simulink model "belt_driven_ergometer"  (R2019b)
settings: Solver=VariableStepAuto  StartTime=0.0  StopTime=10.0  RelTol=1e-3
InitFcn:
  | Kt=0.21
  | rm=0.0135
  | rf=0.15
  | Jm=5.3e-5
  | Jf=2.57e-2
  | Jeq=2.62e-4
  | Jp=5.2e-3
  | Kbelt=8312.1
  | Bbelt=5.96
  | K1=15791
  | K2=251.33
  | N=11.11
  | Ka=2.52e-2
  | Kp=1.664
  | Ki=26.1382
undefined symbols (not defined in the file or in its folder): f, Jeqe, Kte
libraries: powerlib x19, powerlib_extras x3, powerlib_meascontrol x2, simulink x2
settings Model: Creator=李瑾年  LastModifiedBy=李瑾年

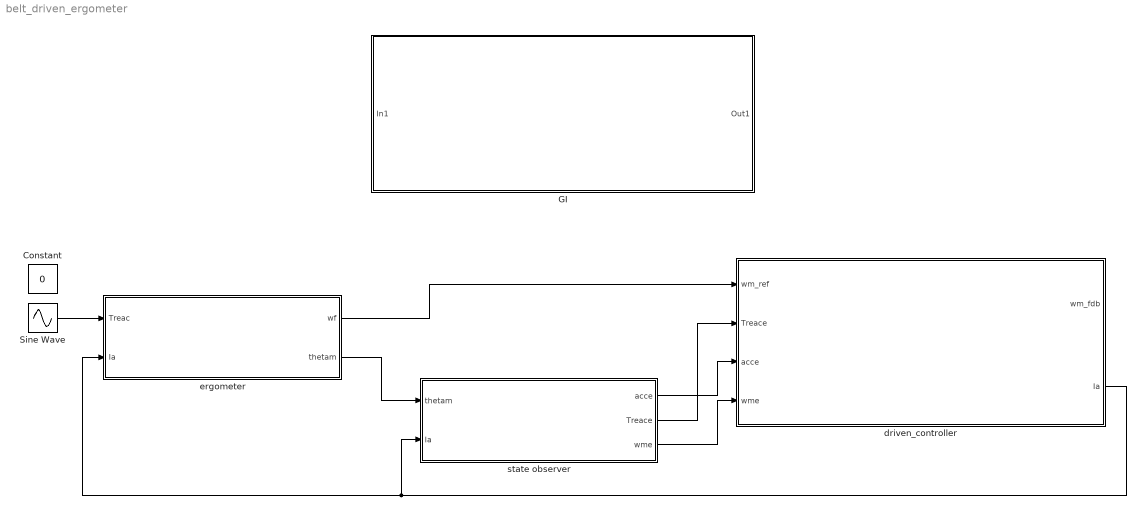
== system belt_driven_ergometer ==
  Constant : Constant  Value=0
  GI : Subsystem
  Sine Wave : Sin  Amplitude=0.5  Bias=-0.5  Frequency=2*pi*f  SampleTime=0
  driven_controller : Subsystem
  ergometer : Subsystem
  state observer : Subsystem
  wires:
  ergometer/1(wf) -> driven_controller/1(wm_ref)
  ergometer/2("thetam  ") -> state observer/1(thetam)
  state observer/2(" Treace ") -> driven_controller/2(Treace)
  state observer/1(" acce") -> driven_controller/3(acce)
  state observer/3(" wme") -> driven_controller/4(wme)
  driven_controller/2(Ia) -> ergometer/2(Ia), state observer/2(Ia)
  Sine Wave/1 -> ergometer/1(Treac)

== system belt_driven_ergometer/GI ==
  In1 : Inport
  Gain3 : Gain  Gain=N*Kt
  Qi Fcn : TransferFcn  Numerator=[15791]  Denominator=[251.33 15791]
  Qo Fcn1 : TransferFcn  Denominator=[0.05 1]
  Sum2 : Sum  Inputs=|+-
  Transfer Fcn : TransferFcn  Numerator=[K1]  Denominator=[1 K2 K1]
  Transfer Fcn1 : TransferFcn  Numerator=[K2 K1]  Denominator=[1 K2 K1]
  phai_I : TransferFcn  Numerator=[Jf rf^2*Bbelt rf^2*Kbelt]  Denominator=[Jp rf^2*Bbelt rf^2*Kbelt]
  Out1 : Outport
  wires:
  Transfer Fcn/1 -> phai_I/1
  Gain3/1 -> Qo Fcn1/1
  Sum2/1 -> Gain3/1  "a"
  Qi Fcn/1 -> Sum2/2
  phai_I/1 -> Sum2/1
  Qo Fcn1/1 -> Out1/1
  In1/1 -> Transfer Fcn1/1, Transfer Fcn/1

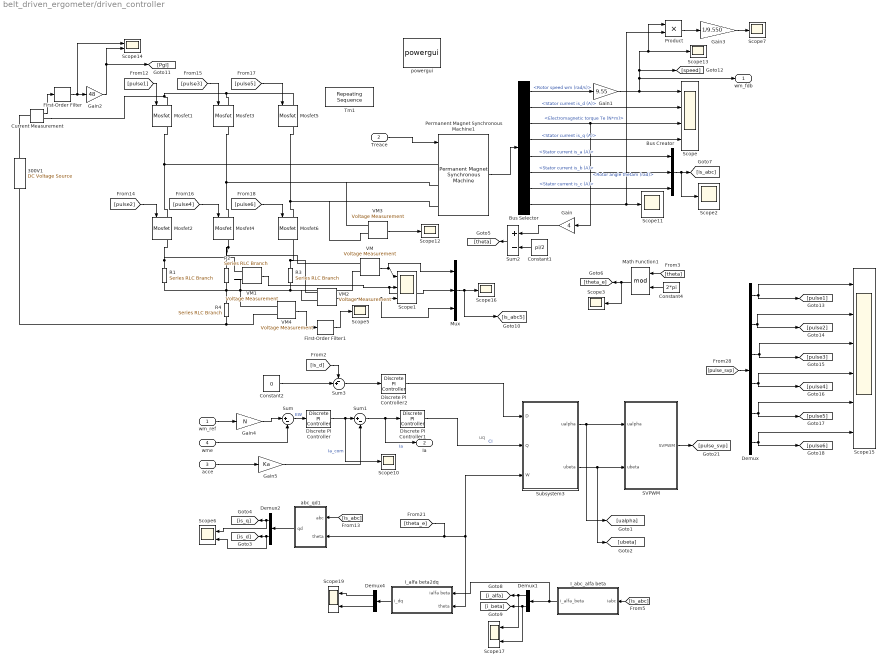
== system belt_driven_ergometer/driven_controller ==
  note: uq
  wm_ref : Inport
  Treace : Inport  Port=2
  acce : Inport  Port=3
  wme : Inport  Port=4
  300V1 : powerlib/Electrical Sources/DC Voltage Source  Amplitude=300  Measurements=Voltage
  Bus Creator : BusCreator  Inputs=3
  Bus Selector : BusSelector  OutputSignals=Rotor speed wm (rad/s),Stator current is_d (A),Rotor angle thetam (rad),Stator current is_q (A),Stator current is_a (A),Stator current is_b (A),Stator current is_c (A),Electromagnetic torque Te (N*m)
  Constant1 : Constant  Value=pi/2
  Constant2 : Constant  Value=0
  Constant4 : Constant  Value=2*pi
  Current Measurement : powerlib/Measurements/Current Measurement  PhasorSimulation=off  OutputType=Complex  PSBequivalent=0
  Demux : Demux  Outputs=6
  Demux1 : Demux  Outputs=2
  Demux2 : Demux  Outputs=2
  Demux4 : Demux  Outputs=2
  Discrete PI Controller : powerlib_extras/Discrete  Control Blocks/Discrete PI Controller  Kp=Kp  Ki=Ki  Par_Limits=[500 -500]  Init=0  Ts=50e-6
      settings: SourceProductName=Simscape Electrical
  Discrete PI Controller1 : powerlib_extras/Discrete  Control Blocks/Discrete PI Controller  Kp=50  Ki=1000  Par_Limits=[1000 -1000]  Init=0  Ts=50e-6
      settings: SourceProductName=Simscape Electrical
  Discrete PI Controller2 : powerlib_extras/Discrete  Control Blocks/Discrete PI Controller  Kp=50  Ki=1000  Par_Limits=[1000 -1000]  Init=0  Ts=50e-6
      settings: SourceProductName=Simscape Electrical
  First-Order Filter : powerlib_meascontrol/Filters/First-Order Filter  FilterType=Lowpass  Tc=0.005  Ts=5e-6  Initialize=off  Vac_Init=[0, 0, 60]  Vdc_Init=0  PlotResponse=off  FreqRange="[0,  200,  1]"
      settings: SourceProductName=Simscape Power Systems
  First-Order Filter1 : powerlib_meascontrol/Filters/First-Order Filter  FilterType=Lowpass  Tc=0.005  Ts=5e-6  Initialize=off  Vac_Init=[0, 0, 60]  Vdc_Init=0  PlotResponse=off  FreqRange="[0,  200,  1]"
      settings: SourceProductName=Simscape Power Systems
  Gain : Gain  Gain=4
  Gain1 : Gain  Gain=9.55
  Gain2 : Gain  Gain=48
  Gain3 : Gain  Gain=1/9.550
  Gain4 : Gain  Gain=N
  Gain5 : Gain  Gain=Ka
  I_abc_alfa beta : Subsystem
  I_alfa beta2dq : Subsystem
  Math Function1 : Math  Operator=mod  SaturateOnIntegerOverflow=on
  Mosfet{1..6} (6 alike) : powerlib/Power Electronics/Mosfet  Ron=0.1  Lon=0  Rd=0.01  Vfd=0  IC=0  Rs=1e5  Cs=inf  Measurements=on
  Mux : Mux  Inputs=3
  Permanent Magnet Synchronous Machine1 : powerlib/Machines/Permanent Magnet Synchronous Machine  NbPhases=3  FluxDistribution=Sinusoidal  RotorType=Round  MechanicalLoad=Torque Tm  PresetModel=No  ShowDetailedParameters=on  MeasurementBus=off  Resistance=0.033  Inductance=8.5e-3  dqInductances=[0.02682 0.02682]  La=0.000805  MachineConstant=Torque Constant (N.m / A_peak)  Flux=0.13847  VoltageCst=100.4591  TorqueCst=0.83079  Flat=120  Mechanical=[0.0001 0.0008 4]  PolePairs=4  InitialConditions=[0,0, 0,0]  InitialConditions5ph=[0 0 0 0 0 0]  RefAngle=90 degrees behind phase A axis (modified Park)  IterativeDiscreteModel=Trapezoidal non iterative  TsBlock=-1  TsPowergui=0
      settings: SourceProductName=Simscape Power Systems
  Product : Product
  R1 : powerlib/Elements/Series RLC Branch  LConnTagsString=__new0  RConnTagsString=__new0  BranchType=R  Resistance=0.003  Inductance=1e-3  SetiL0=off  InitialCurrent=0  Capacitance=1e-6  Setx0=off  InitialVoltage=0  Measurements=None
  R2 : powerlib/Elements/Series RLC Branch  LConnTagsString=__new0  RConnTagsString=__new0  BranchType=R  Resistance=0.003  Inductance=1e-3  SetiL0=off  InitialCurrent=0  Capacitance=1e-6  Setx0=off  InitialVoltage=0  Measurements=None
  R3 : powerlib/Elements/Series RLC Branch  LConnTagsString=__new0  RConnTagsString=__new0  BranchType=R  Resistance=0.003  Inductance=1e-3  SetiL0=off  InitialCurrent=0  Capacitance=1e-6  Setx0=off  InitialVoltage=0  Measurements=None
  R4 : powerlib/Elements/Series RLC Branch  LConnTagsString=__new0  RConnTagsString=__new0  BranchType=R  Resistance=0.002  Inductance=1e-3  SetiL0=off  InitialCurrent=0  Capacitance=1e-6  Setx0=off  InitialVoltage=0  Measurements=None
  SVPWM : Subsystem
  Scope : Scope  NumInputPorts=4
  Scope1 : Scope  NumInputPorts=3
  Scope{2..3,5,7,10..13,16} (9 alike) : Scope
  Scope{6,14,17,19} (4 alike) : Scope  NumInputPorts=2
  Scope15 : Scope  NumInputPorts=6
  Subsystem3 : Subsystem
  Sum : Sum  Inputs=|+-
  Sum1 : Sum  Inputs=|+-
  Sum2 : Sum  Inputs=+-  SaturateOnIntegerOverflow=on  InputSameDT=on  OutDataTypeStr=Inherit: Same as first input
  Sum3 : Sum  Inputs=-+|
  Tm1 : simulink/Sources/Repeating Sequence  rep_seq_t="[0  0.3    ]"  rep_seq_y="[ 40  70 ]"
  VM{,1..4} (5 alike) : powerlib/Measurements/Voltage Measurement  PhasorSimulation=off  OutputType=Complex  PSBequivalent=0
  abc_qd1 : Subsystem
  powergui : powerlib/powergui  SimulationMode=Discrete  SampleTime=5e-6  frequency=60  Iterations=50  frequencyindice=0  Pbase=100e6  ErrMax=1e-4  UnitsV=kV  UnitsW=MW  buscounter=0  FunctionMessages=off  echomessages=off  EnableUseOfTLC=off  CurrentSourceSwitches=off  DisableSnubberDevices=off  DisableRonSwitches=off  DisableVfSwitches=off  DisplayEquations=off  AutomaticDiscreteSolvers=off  SolverType=Tustin  Interpol=off  ExternalGateDelay=off  methode=off  Ts=0  x0status=blocks  SPID=off  SwTol=0  HookPort=off  NonlinearTolerance=1e-4  nMaxIteration=100  ContinueOnMaxIteration=off  RestoreLinks=warning  ResistiveCurrentMeasurement=off  Frange=[0:2:500]  Ylog=off  Xlog=on  ShowGrid=off  save=off  variable=ZData  structure=0  ZoomFFT=on  StartTime=0.0  cycles=1  DisplayStyle=1  fundamental=60  FreqAxis=off  MaxFrequency=1000  frequencyindicesteady=1  RmsSteady=1  display=off
  wm_fdb : Outport
  Ia : Outport  Port=2
  wires:
  I_alfa beta2dq/1(i_dq) -> Demux4/1
  abc_qd1/1(qd) -> Demux2/1
  Product/1 -> Gain3/1
  [pulse4] -> Mosfet4/1
  [pulse5] -> Mosfet5/1
  VM2/1 -> Mux/3, Scope1/3
  [pulse2] -> Mosfet2/1
  [pulse3] -> Mosfet3/1
  Permanent Magnet Synchronous Machine1/1 -> Bus Selector/1
  Demux1/2 -> [i_beta], Scope17/2
  Demux/3 -> [pulse3], Scope15/3
  Demux4/2 -> Scope19/2
  [pulse1] -> Mosfet1/1
  VM1/1 -> Mux/2, Scope1/2
  First-Order Filter1/1 -> Scope5/1
  Bus Selector/8 -> Product/2, Scope11/1  "<Electromagnetic torque Te (N*m)>"
  VM3/1 -> Scope12/1
  Discrete PI Controller1/1 -> Subsystem3/2(Q)  "CI"
  Demux/2 -> [pulse2], Scope15/2
  Subsystem3/2(ubeta) -> [ubeta], SVPWM/2(ubeta)
  [theta_e] -> I_alfa beta2dq/2(theta), Subsystem3/3(W), abc_qd1/2(theta)
  Subsystem3/1(ualpha) -> [ualpha], SVPWM/1(ualpha)
  [pulse6] -> Mosfet6/1
  Demux/4 -> [pulse4], Scope15/4
  Bus Creator/1 -> Scope2/1, [is_abc]
  Mux/1 -> [is_abcS], Scope16/1
  Bus Selector/4 -> Scope/4  "<Stator current is_q (A)>"
  wme/1 -> Sum/2
  Demux1/1 -> [i_alfa], Scope17/1
  [is_d] -> Sum3/1
  [is_abc] -> I_abc_alfa beta/1(iabc)
  VM/1 -> Mux/1, Scope1/1
  I_abc_alfa beta/1(i_alfa_beta) -> I_alfa beta2dq/1(ialfa beta), Demux1/1
  Demux/1 -> [pulse1], Scope15/1
  Gain2/1 -> [Pgl], Scope14/2
  Current Measurement/1 -> First-Order Filter/1
  Demux4/1 -> Scope19/1
  SVPWM/1(SVPWM) -> [pulse_svp]
  VM4/1 -> First-Order Filter1/1
  Gain3/1 -> Scope7/1
  First-Order Filter/1 -> Scope14/1, Gain2/1
  Math Function1/1 -> Scope3/1, [theta_e]
  Bus Selector/6 -> Bus Creator/2  "<Stator current is_b (A)>"
  Demux/6 -> [pulse6], Scope15/6
  Constant4/1 -> Math Function1/2
  Sum2/1 -> [theta]
  Demux2/2 -> Scope6/2, [is_d]
  Sum3/1 -> Discrete PI Controller2/1
  Bus Selector/2 -> Scope/2  "<Stator current is_d (A)>"
  Gain1/1 -> Scope/1, Product/1, Scope13/1, [speed], wm_fdb/1
  [theta] -> Math Function1/1
  Demux2/1 -> Scope6/1, [is_q]
  [is_abc] -> abc_qd1/1(abc)
  Sum1/1 -> Ia/1, Discrete PI Controller1/1  "Ia"
  Constant2/1 -> Sum3/2
  Bus Selector/5 -> Bus Creator/1  "<Stator current is_a (A)>"
  [pulse_svp] -> Demux/1
  Bus Selector/3 -> Gain/1, Scope/3  "<Rotor angle thetam (rad)>"
  Gain5/1 -> Sum1/2
  Discrete PI Controller/1 -> Scope10/1, Sum1/1  "Ia_com"
  Constant1/1 -> Sum2/2
  Bus Selector/1 -> Gain1/1  "<Rotor speed wm (rad/s)>"
  Bus Selector/7 -> Bus Creator/3  "<Stator current is_c (A)>"
  Discrete PI Controller2/1 -> Subsystem3/1(D)
  Gain/1 -> Sum2/1
  Sum/1 -> Discrete PI Controller/1  "EW"
  Demux/5 -> [pulse5], Scope15/5
  Treace/1 -> Permanent Magnet Synchronous Machine1/1
  wm_ref/1 -> Gain4/1
  Gain4/1 -> Sum/1
  acce/1 -> Gain5/1
  connections:
  VM4/LConn2 -- R4/RConn1 -- 300V1/LConn1
  Mosfet4/RConn1 -- VM/LConn1 -- R2/LConn1
  R3/RConn1 -- R1/RConn1 -- R4/LConn1 -- R2/RConn1 -- VM4/LConn1 -- VM1/LConn2 -- VM2/LConn2 -- VM/LConn2
  Mosfet6/LConn1 -- Mosfet5/RConn1 -- Permanent Magnet Synchronous Machine1/LConn3 -- VM3/LConn2
  Current Measurement/RConn1 -- Mosfet1/LConn1 -- Mosfet5/LConn1 -- Mosfet3/LConn1
  R1/LConn1 -- Mosfet2/RConn1 -- VM1/LConn1
  VM2/LConn1 -- R3/LConn1 -- Mosfet6/RConn1
  Mosfet4/LConn1 -- Permanent Magnet Synchronous Machine1/LConn2 -- VM3/LConn1 -- Mosfet3/RConn1
  Mosfet2/LConn1 -- Permanent Magnet Synchronous Machine1/LConn1 -- Mosfet1/RConn1
  Current Measurement/LConn1 -- 300V1/RConn1

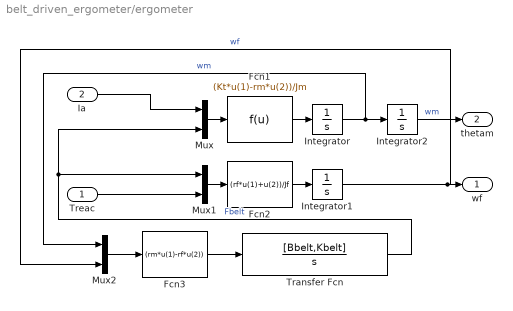
== system belt_driven_ergometer/ergometer ==
  Treac : Inport
  Ia : Inport  Port=2
  Fcn1 : Fcn  Expr=(Kt*u(1)-rm*u(2))/Jm
  Fcn2 : Fcn  Expr=(rf*u(1)+u(2))/Jf
  Fcn3 : Fcn  Expr=(rm*u(1)-rf*u(2))
  Integrator : Integrator
  Integrator1 : Integrator
  Integrator2 : Integrator
  Mux : Mux  Inputs=2
  Mux1 : Mux  Inputs=2
  Mux2 : Mux  Inputs=2
  Transfer Fcn : TransferFcn  Numerator=[Bbelt,Kbelt]  Denominator=[1 0]
  wf : Outport
  "thetam  " : Outport  Port=2
  wires:
  Mux/1 -> Fcn1/1
  Fcn2/1 -> Integrator1/1
  Treac/1 -> Mux1/2
  Ia/1 -> Mux/1
  Fcn3/1 -> Transfer Fcn/1
  Integrator1/1 -> Mux2/2, wf/1  "wf"
  Transfer Fcn/1 -> Mux1/1, Mux/2  "Fbelt"
  Integrator/1 -> Integrator2/1, Mux2/1  "wm"
  Mux2/1 -> Fcn3/1
  Mux1/1 -> Fcn2/1
  Fcn1/1 -> Integrator/1
  Integrator2/1 -> "thetam  "/1  "wm"

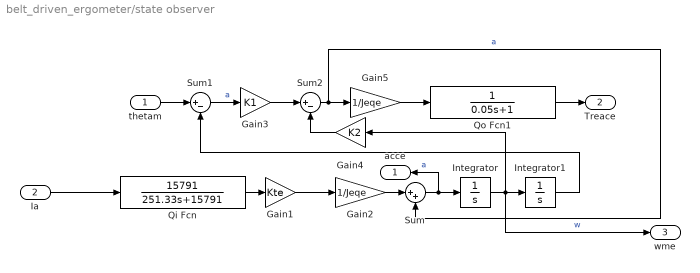
== system belt_driven_ergometer/state observer ==
  thetam : Inport
  Ia : Inport  Port=2
  Gain1 : Gain  Gain=Kte
  Gain2 : Gain  Gain=1/Jeqe
  Gain3 : Gain  Gain=K1
  Gain4 : Gain  Gain=K2
  Gain5 : Gain  Gain=1/Jeqe
  Integrator : Integrator
  Integrator1 : Integrator
  Qi Fcn : TransferFcn  Numerator=[15791]  Denominator=[251.33 15791]
  Qo Fcn1 : TransferFcn  Denominator=[0.05 1]
  Sum : Sum  Inputs=|++
  Sum1 : Sum  Inputs=|+-
  Sum2 : Sum  Inputs=|+-
  " acce" : Outport
  " Treace " : Outport  Port=2
  " wme" : Outport  Port=3
  wires:
  Ia/1 -> Qi Fcn/1
  Qi Fcn/1 -> Gain1/1
  Gain1/1 -> Gain2/1
  Gain2/1 -> Sum/1
  Sum/1 -> " acce"/1, Integrator/1  "a"
  Integrator/1 -> " wme"/1, Gain4/1, Integrator1/1  "w"
  thetam/1 -> Sum1/1
  Integrator1/1 -> Sum1/2
  Sum1/1 -> Gain3/1  "a"
  Gain3/1 -> Sum2/1
  Gain4/1 -> Sum2/2
  Sum2/1 -> Gain5/1, Sum/2  "a"
  Gain5/1 -> Qo Fcn1/1
  Qo Fcn1/1 -> " Treace "/1

== system belt_driven_ergometer/driven_controller/I_abc_alfa beta ==
  iabc : Inport
  Fcn : Fcn  Expr=(2*u(1)-u(2)-u(3))/3
  Fcn1 : Fcn  Expr=(u(2)-u(3))/(3^(1/2))
  Mux2 : Mux  Inputs=2
  i_alfa_beta : Outport  VectorParamsAs1DForOutWhenUnconnected=off
  wires:
  Fcn1/1 -> Mux2/2
  Fcn/1 -> Mux2/1
  Mux2/1 -> i_alfa_beta/1
  iabc/1 -> Fcn1/1, Fcn/1

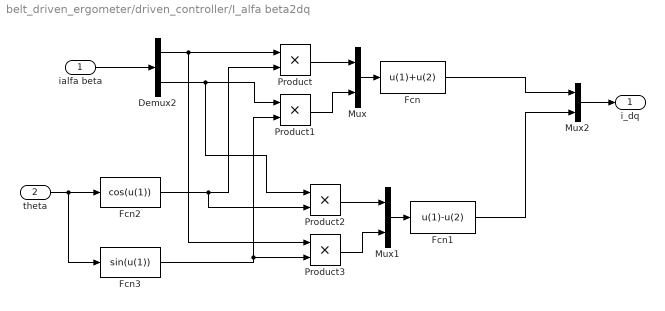
== system belt_driven_ergometer/driven_controller/I_alfa beta2dq ==
  ialfa beta : Inport
  theta : Inport  Port=2
  Demux2 : Demux  Outputs=2
  Fcn : Fcn  Expr=u(1)+u(2)
  Fcn1 : Fcn  Expr=u(1)-u(2)
  Fcn2 : Fcn  Expr=cos(u(1))
  Fcn3 : Fcn  Expr=sin(u(1))
  Mux : Mux  Inputs=2
  Mux1 : Mux  Inputs=2
  Mux2 : Mux  Inputs=2
  Product{,1..3} (4 alike) : Product
  i_dq : Outport  VectorParamsAs1DForOutWhenUnconnected=off
  wires:
  Fcn/1 -> Mux2/1
  Mux2/1 -> i_dq/1
  theta/1 -> Fcn3/1, Fcn2/1
  ialfa beta/1 -> Demux2/1
  Demux2/1 -> Product3/1, Product/1
  Demux2/2 -> Product2/1, Product1/1
  Fcn2/1 -> Product2/2, Product/2
  Fcn3/1 -> Product3/2, Product1/2
  Product1/1 -> Mux/2
  Product/1 -> Mux/1
  Mux/1 -> Fcn/1
  Fcn1/1 -> Mux2/2
  Product3/1 -> Mux1/2
  Product2/1 -> Mux1/1
  Mux1/1 -> Fcn1/1

== system belt_driven_ergometer/driven_controller/SVPWM ==
  ualpha : Inport
  ubeta : Inport  Port=2
  Constant : Constant  Value=300
  Constant1 : Constant  Value=0.0002
  Subsystem : Subsystem
  Subsystem1 : Subsystem
  Subsystem2 : Subsystem
  Subsystem3 : Subsystem
  Subsystem4 : Subsystem
  SVPWM : Outport  VectorParamsAs1DForOutWhenUnconnected=off
  wires:
  ualpha/1 -> Subsystem/1(1), Subsystem1/1(1)
  Subsystem1/1(a) -> Subsystem2/1(a)
  Subsystem1/2(b) -> Subsystem2/2(b)
  Subsystem1/3(c) -> Subsystem2/3(c)
  Subsystem/1(s) -> Subsystem2/4(s), Subsystem3/1(s)
  Subsystem2/1(1) -> Subsystem3/2(T1)
  Subsystem2/2(2) -> Subsystem3/3(T2)
  Subsystem3/1(1) -> Subsystem4/1(A)
  Subsystem3/2(2) -> Subsystem4/2(B)
  Subsystem3/3(3) -> Subsystem4/3(C)
  Constant/1 -> Subsystem1/4(U)
  Constant1/1 -> Subsystem2/5(T3), Subsystem1/3(3), Subsystem3/4(T3)
  Subsystem4/1(SVPWM) -> SVPWM/1
  ubeta/1 -> Subsystem1/2(2), Subsystem/2(2)

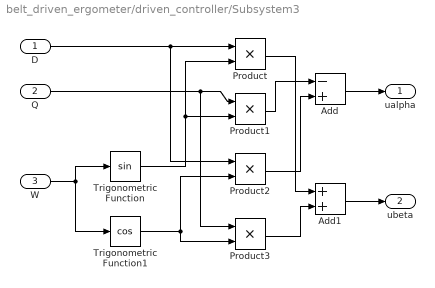
== system belt_driven_ergometer/driven_controller/Subsystem3 ==
  D : Inport
  Q : Inport  Port=2
  W : Inport  Port=3
  Add : Sum  Inputs=-+
  Add1 : Sum
  Product{,1..3} (4 alike) : Product  RndMeth=Zero
  Trigonometric Function : Trigonometry
  Trigonometric Function1 : Trigonometry  Operator=cos
  ualpha : Outport  VectorParamsAs1DForOutWhenUnconnected=off
  ubeta : Outport  Port=2  VectorParamsAs1DForOutWhenUnconnected=off
  wires:
  W/1 -> Trigonometric Function/1, Trigonometric Function1/1
  Trigonometric Function/1 -> Product/2, Product1/2
  Trigonometric Function1/1 -> Product2/2, Product3/2
  D/1 -> Product/1, Product2/1
  Q/1 -> Product1/1, Product3/1
  Add/1 -> ualpha/1
  Add1/1 -> ubeta/1
  Product2/1 -> Add/2
  Product1/1 -> Add/1
  Product/1 -> Add1/1
  Product3/1 -> Add1/2

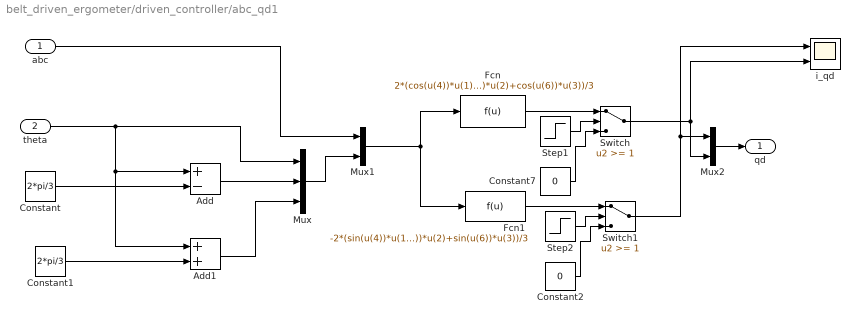
== system belt_driven_ergometer/driven_controller/abc_qd1 ==
  abc : Inport
  theta : Inport  Port=2
  Add : Sum  Inputs=+-
  Add1 : Sum
  Constant : Constant  Value=2*pi/3
  Constant1 : Constant  Value=2*pi/3
  Constant2 : Constant  Value=0
  Constant7 : Constant  Value=0
  Fcn : Fcn  Expr=2*(cos(u(4))*u(1)+cos(u(5))*u(2)+cos(u(6))*u(3))/3
  Fcn1 : Fcn  Expr=-2*(sin(u(4))*u(1)+sin(u(5))*u(2)+sin(u(6))*u(3))/3
  Mux : Mux  Inputs=3
  Mux1 : Mux  Inputs=2
  Mux2 : Mux  Inputs=2
  Step1 : Step  Time=0.0001  SampleTime=0
  Step2 : Step  Time=0.0001  SampleTime=0
  Switch : Switch  Threshold=1
  Switch1 : Switch  Threshold=1
  "i_qd " : Scope  NumInputPorts=2
  qd : Outport  VectorParamsAs1DForOutWhenUnconnected=off
  wires:
  Switch1/1 -> "i_qd "/1, Mux2/1
  Constant2/1 -> Switch1/3
  Step2/1 -> Switch1/2
  Fcn1/1 -> Switch1/1
  Constant7/1 -> Switch/3
  Step1/1 -> Switch/2
  Switch/1 -> "i_qd "/2, Mux2/2
  Fcn/1 -> Switch/1
  Mux2/1 -> qd/1
  Mux1/1 -> Fcn1/1, Fcn/1
  abc/1 -> Mux1/1
  Mux/1 -> Mux1/2
  Add1/1 -> Mux/3
  Add/1 -> Mux/2
  theta/1 -> Add/1, Add1/1, Mux/1
  Constant/1 -> Add/2
  Constant1/1 -> Add1/2

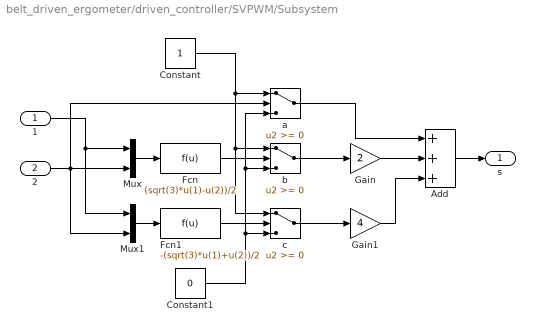
== system belt_driven_ergometer/driven_controller/SVPWM/Subsystem ==
  1 : Inport
  2 : Inport  Port=2
  Add : Sum  Inputs=+++
  Constant : Constant
  Constant1 : Constant  Value=0
  Fcn : Fcn  Expr=(sqrt(3)*u(1)-u(2))/2
  Fcn1 : Fcn  Expr=-(sqrt(3)*u(1)+u(2))/2
  Gain : Gain  Gain=2
  Gain1 : Gain  Gain=4
  Mux : Mux  Inputs=2
  Mux1 : Mux  Inputs=2
  a : Switch
  b : Switch
  c : Switch
  s : Outport  VectorParamsAs1DForOutWhenUnconnected=off
  wires:
  1/1 -> Mux/1, Mux1/1
  Constant/1 -> a/1, b/1, c/1
  2/1 -> Mux/2, Mux1/2, a/2
  Mux/1 -> Fcn/1
  Fcn/1 -> b/2
  Mux1/1 -> Fcn1/1
  Fcn1/1 -> c/2
  Constant1/1 -> c/3, b/3, a/3
  b/1 -> Gain/1
  c/1 -> Gain1/1
  Gain/1 -> Add/2
  a/1 -> Add/1
  Gain1/1 -> Add/3
  Add/1 -> s/1

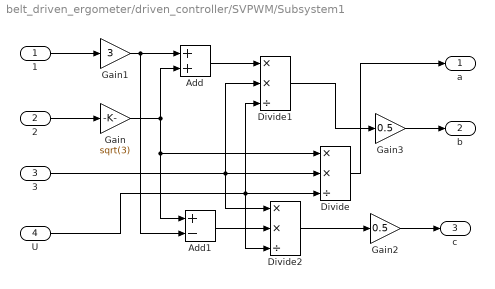
== system belt_driven_ergometer/driven_controller/SVPWM/Subsystem1 ==
  1 : Inport
  2 : Inport  Port=2
  3 : Inport  Port=3
  U : Inport  Port=4
  Add : Sum
  Add1 : Sum  Inputs=+-
  Divide : Product  Inputs=**/
  Divide1 : Product  Inputs=**/
  Divide2 : Product  Inputs=**/
  Gain : Gain  Gain=sqrt(3)
  Gain1 : Gain  Gain=3
  Gain2 : Gain  Gain=0.5
  Gain3 : Gain  Gain=0.5
  a : Outport  VectorParamsAs1DForOutWhenUnconnected=off
  b : Outport  Port=2  VectorParamsAs1DForOutWhenUnconnected=off
  c : Outport  Port=3  VectorParamsAs1DForOutWhenUnconnected=off
  wires:
  2/1 -> Gain/1
  Gain/1 -> Add/2, Divide/1, Add1/1
  3/1 -> Divide/2, Divide1/2, Divide2/1
  U/1 -> Divide/3, Divide1/3, Divide2/3
  1/1 -> Gain1/1
  Gain1/1 -> Add/1, Add1/2
  Add/1 -> Divide1/1
  Add1/1 -> Divide2/2
  Divide2/1 -> Gain2/1
  Gain2/1 -> c/1
  Divide/1 -> a/1
  Divide1/1 -> Gain3/1
  Gain3/1 -> b/1

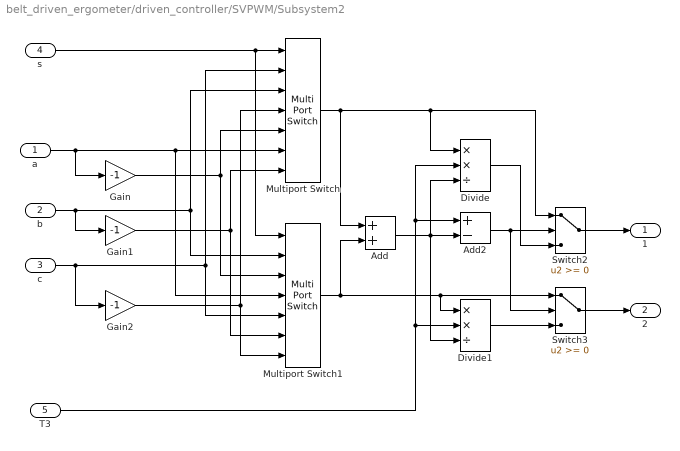
== system belt_driven_ergometer/driven_controller/SVPWM/Subsystem2 ==
  a : Inport
  b : Inport  Port=2
  c : Inport  Port=3
  s : Inport  Port=4
  T3 : Inport  Port=5
  Add : Sum
  Add2 : Sum  Inputs=+-
  Divide : Product  Inputs=**/
  Divide1 : Product  Inputs=**/
  Gain : Gain  Gain=-1
  Gain1 : Gain  Gain=-1
  Gain2 : Gain  Gain=-1
  Multiport Switch : MultiPortSwitch  Inputs=6  DiagnosticForDefault=None  SampleTime=5e-6
  Multiport Switch1 : MultiPortSwitch  Inputs=6  DiagnosticForDefault=None  SampleTime=5e-6
  Switch2 : Switch
  Switch3 : Switch
  1 : Outport  VectorParamsAs1DForOutWhenUnconnected=off
  2 : Outport  Port=2  VectorParamsAs1DForOutWhenUnconnected=off
  wires:
  s/1 -> Multiport Switch/1, Multiport Switch1/1
  b/1 -> Gain1/1, Multiport Switch/3, Multiport Switch1/2
  a/1 -> Gain/1, Multiport Switch/6, Multiport Switch1/4
  c/1 -> Gain2/1, Multiport Switch/2, Multiport Switch1/5
  Multiport Switch/1 -> Add/1, Divide/1, Switch2/1
  Multiport Switch1/1 -> Add/2, Switch3/1, Divide1/1
  T3/1 -> Divide1/2, Divide/2, Add2/1
  Add2/1 -> Switch2/2, Switch3/2
  Divide/1 -> Switch2/3
  Divide1/1 -> Switch3/3
  Switch3/1 -> 2/1
  Switch2/1 -> 1/1
  Add/1 -> Divide/3, Divide1/3, Add2/2
  Gain1/1 -> Multiport Switch1/6, Multiport Switch/7
  Gain2/1 -> Multiport Switch/4, Multiport Switch1/7
  Gain/1 -> Multiport Switch/5, Multiport Switch1/3

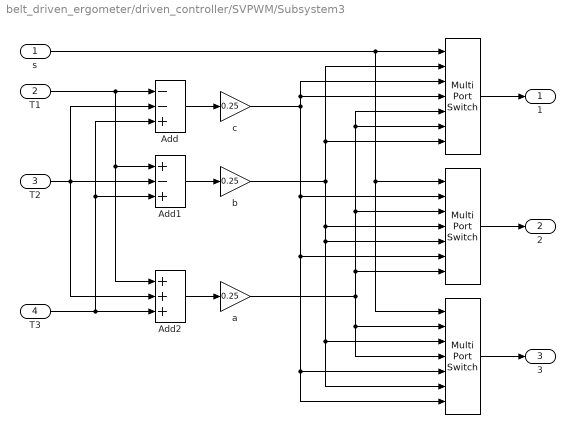
== system belt_driven_ergometer/driven_controller/SVPWM/Subsystem3 ==
  s : Inport
  T1 : Inport  Port=2
  T2 : Inport  Port=3
  T3 : Inport  Port=4
  " " : MultiPortSwitch  Inputs=6  DiagnosticForDefault=None
  "  " : MultiPortSwitch  Inputs=6  DiagnosticForDefault=None
  "    " : MultiPortSwitch  Inputs=6  DiagnosticForDefault=None
  Add : Sum  Inputs=--+
  Add1 : Sum  Inputs=+-+
  Add2 : Sum  Inputs=+++
  a : Gain  Gain=0.25
  b : Gain  Gain=0.25
  c : Gain  Gain=0.25
  1 : Outport  VectorParamsAs1DForOutWhenUnconnected=off
  2 : Outport  Port=2  VectorParamsAs1DForOutWhenUnconnected=off
  3 : Outport  Port=3  VectorParamsAs1DForOutWhenUnconnected=off
  wires:
  s/1 -> "  "/1, " "/1, "    "/1
  T1/1 -> Add/1, Add1/1, Add2/1
  T2/1 -> Add/2, Add1/2, Add2/2
  T3/1 -> Add/3, Add1/3, Add2/3
  Add/1 -> c/1
  Add1/1 -> b/1
  Add2/1 -> a/1
  "  "/1 -> 1/1
  " "/1 -> 2/1
  "    "/1 -> 3/1
  b/1 -> "  "/7, "  "/2, " "/4, " "/5, "    "/3, "    "/6
  c/1 -> " "/2, " "/6, "    "/5, "    "/7, "  "/4, "  "/3
  a/1 -> "  "/5, "  "/6, " "/3, " "/7, "    "/2, "    "/4

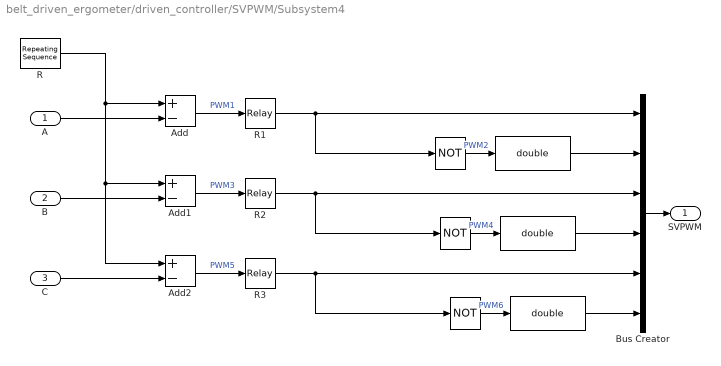
== system belt_driven_ergometer/driven_controller/SVPWM/Subsystem4 ==
  A : Inport
  B : Inport  Port=2
  C : Inport  Port=3
  " " : Logic  Operator=NOT  AllPortsSameDT=off  OutDataTypeStr=boolean
  "  " : DataTypeConversion  OutDataTypeStr=double
  "   " : Logic  Operator=NOT  AllPortsSameDT=off  OutDataTypeStr=boolean
  "     " : DataTypeConversion  OutDataTypeStr=double
  "       " : Logic  Operator=NOT  AllPortsSameDT=off  OutDataTypeStr=boolean
  "         " : DataTypeConversion  OutDataTypeStr=double
  Add : Sum  Inputs=+-
  Add1 : Sum  Inputs=+-
  Add2 : Sum  Inputs=+-
  Bus Creator : BusCreator  Inputs=6
  R : simulink/Sources/Repeating Sequence  rep_seq_t="[0  0.0001  0.0002]"  rep_seq_y="[0  0.0001  0]"
  R1 : Relay
  R2 : Relay
  R3 : Relay
  SVPWM : Outport  VectorParamsAs1DForOutWhenUnconnected=off
  wires:
  A/1 -> Add/2
  B/1 -> Add1/2
  C/1 -> Add2/2
  R/1 -> Add/1, Add1/1, Add2/1
  Add/1 -> R1/1  "PWM1"
  Add1/1 -> R2/1  "PWM3"
  Add2/1 -> R3/1  "PWM5"
  " "/1 -> "  "/1  "PWM2"
  "   "/1 -> "     "/1  "PWM4"
  "       "/1 -> "         "/1  "PWM6"
  Bus Creator/1 -> SVPWM/1
  R1/1 -> Bus Creator/1, " "/1
  R3/1 -> Bus Creator/5, "       "/1
  R2/1 -> Bus Creator/3, "   "/1
  "         "/1 -> Bus Creator/6
  "     "/1 -> Bus Creator/4
  "  "/1 -> Bus Creator/2
